simulink model "stm32f0_ccp_sensor"  (Simulink 7.3)
settings: Solver=ode3  SolverMode=SingleTasking  StartTime=0.0  StopTime=10.0  RelTol=1e-3
PreLoadFcn:
  | waijung.modelPreload; % Required for working with Waijung Blockset. Do not remove.
undefined symbols (not defined in the file): ARM, LQFP48, MDK, STM32F072CB
libraries: simulink x216, waijung_soft_i2c_lib x28, waijung_addon_module x12, stm32f0_flash_lib x10, stm32f0_can_lib x3, stm32f0_reset_lib x1, waijung_crc_lib x1, stm32f0_boot_lib x1, stm32f0_device_config_lib x1
(part 5 of 6)

== system stm32f0_ccp_sensor/CCP Handler/Command Processing/BUILD_CHKSUM/BUILD_CHKSUM Handler/Subsystem/While Iterator Subsystem ==
  Address : Inport  OutDataType=fixdt(1, 16)  OutScaling=2^0
  Size : Inport  Port=2  OutDataType=fixdt(1, 16)  OutScaling=2^0
  Add : Sum  OutDataType=fixdt(1, 16)  OutScaling=2^-10
  Add1 : Sum  OutDataType=fixdt(1, 16)  OutScaling=2^-10
  Bitwise Operator : simulink/Logic and Bit Operations/Bitwise Operator  logicop=AND  UseBitMask=on  BitMask=hex2dec('01FFFFFF')  BitMaskRealWorld=Stored Integer
  Bitwise Operator1 : simulink/Logic and Bit Operations/Bitwise Operator  logicop=AND  UseBitMask=on  BitMask=hex2dec('0001FFFF')  BitMaskRealWorld=Stored Integer
  Compare To Zero : simulink/Logic and Bit Operations/Compare To Zero  SystemSampleTime=-1  relop===  LogicOutDataTypeMode=uint8  ZeroCross=off
  Initial : Constant  Value=0  OutDataTypeMode=uint32  OutDataType=fixdt(1, 16)  OutScaling=2^0  OutDataTypeStr=uint32
  Initial1 : Constant  Value=hex2dec('FFFFFFFF')  OutDataTypeMode=uint32  OutDataType=fixdt(1, 16)  OutScaling=2^0  OutDataTypeStr=uint32
  Memory : Memory  InheritSampleTime=on  LinearizeMemory=on
  Memory1 : Memory  InheritSampleTime=on  LinearizeMemory=on
  Relational Operator : RelationalOperator  Operator=>  LogicOutDataTypeMode=boolean  LogicDataType=fixdt(0, 8)  OutDataTypeStr=boolean
  Step : Constant  Value=4  OutDataTypeMode=uint32  OutDataType=fixdt(1, 16)  OutScaling=2^0  OutDataTypeStr=uint32
  Subsystem : Subsystem
  Switch : Switch  Criteria=u2 ~= 0  OutDataType=fixdt(1, 16)  OutScaling=2^0
  Switch1 : Switch  Criteria=u2 ~= 0  OutDataType=fixdt(1, 16)  OutScaling=2^0
  While Iterator : WhileIterator  MaxIters=-1  WhileBlockType=do-while
  CRC : Outport  OutDataType=fixdt(1, 16)  OutScaling=2^0
  wires:
  Initial/1 -> Switch/3
  Add1/1 -> Switch/1
  Relational Operator/1 -> Switch/2, While Iterator/1, Subsystem/Enable
  Switch/1 -> Memory/1
  Size/1 -> Relational Operator/1
  Step/1 -> Add1/2
  Add/1 -> Bitwise Operator/1
  Memory/1 -> Add/2, Relational Operator/2, Add1/1, Compare To Zero/1
  Address/1 -> Bitwise Operator1/1
  Compare To Zero/1 -> Switch1/2
  Initial1/1 -> Switch1/1
  Switch1/1 -> Subsystem/1(In1)
  Subsystem/1(Out1) -> Memory1/1, CRC/1
  Memory1/1 -> Switch1/3
  Bitwise Operator/1 -> Subsystem/2(In2)
  Bitwise Operator1/1 -> Add/1

== system stm32f0_ccp_sensor/CCP Handler/Command Processing/CLEAR_MEMORY/CLEAR_MEMORY Handler/Flash Erase/While Iterator Subsystem ==
  Address : Inport  OutDataType=fixdt(1, 16)  OutScaling=2^0
  Size : Inport  Port=2  OutDataType=fixdt(1, 16)  OutScaling=2^0
  Add : Sum  OutDataType=fixdt(1, 16)  OutScaling=2^-10
  Add1 : Sum  OutDataType=fixdt(1, 16)  OutScaling=2^-10
  Bitwise Operator : simulink/Logic and Bit Operations/Bitwise Operator  logicop=AND  UseBitMask=on  BitMask=hex2dec('0000FFFF')  BitMaskRealWorld=Stored Integer
  Initial : Constant  Value=0  OutDataTypeMode=uint32  OutDataType=fixdt(1, 16)  OutScaling=2^0  OutDataTypeStr=uint32
  Memory : Memory  InheritSampleTime=on  LinearizeMemory=on
  Relational Operator : RelationalOperator  Operator=>  LogicOutDataTypeMode=boolean  LogicDataType=fixdt(0, 8)  OutDataTypeStr=boolean
  Step : Constant  Value=2048  OutDataTypeMode=uint32  OutDataType=fixdt(1, 16)  OutScaling=2^0  OutDataTypeStr=uint32
  Subsystem : Subsystem
  Switch : Switch  Criteria=u2 ~= 0  OutDataType=fixdt(1, 16)  OutScaling=2^0
  While Iterator : WhileIterator  MaxIters=-1  WhileBlockType=do-while
  Sta : Outport  OutDataType=fixdt(1, 16)  OutScaling=2^0
  wires:
  Bitwise Operator/1 -> Subsystem/1(Address)
  Subsystem/1(Sta) -> Sta/1
  Address/1 -> Add/1
  Memory/1 -> Add1/1, Relational Operator/2, Add/2
  Add/1 -> Bitwise Operator/1
  Step/1 -> Add1/2
  Size/1 -> Relational Operator/1
  Switch/1 -> Memory/1
  Relational Operator/1 -> Switch/2, While Iterator/1, Subsystem/Enable
  Add1/1 -> Switch/1
  Initial/1 -> Switch/3

== system stm32f0_ccp_sensor/CCP Handler/Command Processing/PROGRAM/ PROGRAM_6/PROGRAM/PROGRAM_6 Handler/EEPROM Program/Subsystem ==
  SlaveAddr : Inport
  Offset : Inport  Port=2
  D0 : Inport  Port=3
  Enable : EnablePort
  Compare To Zero : simulink/Logic and Bit Operations/Compare To Zero  SystemSampleTime=-1  relop===  LogicOutDataTypeMode=uint8  ZeroCross=off
  Soft I2C Master Read/Write : waijung_soft_i2c_lib/Soft I2C Master Read//Write  conf=ReadWrite  targetname=stm32f0  module=1  transfer=Blocking  clk=100  timeout=25  sdapins={'A4','A6'}  sclpins='A5'  writecount=2  readcount=0  waittime=5  forcestop=off  portpinstr=0  sampletime=inf  blockid=CCPHandlerCommandProcessingPROGRAMPROGRAM_6PROGRAMPROGRAM_6HandlerEEPROMProgramSubsystemSoftI2CMasterReadWrite  inputporttype=[3 3 3]  inputportwidth=[]  inputportlabel={'SlvAddr' 'Wr0 (uint8)' 'Wr1 (uint8)'}  outputporttype=[3]  outputportwidth=[1]  outputportlabel={'Status'}  compat=0  optionstring="[\"1\",\"2\",\"0\",\"5\",\"off\",\"1\"]"
  Success : Outport
  wires:
  SlaveAddr/1 -> Soft I2C Master Read/Write/1
  Offset/1 -> Soft I2C Master Read/Write/2
  Soft I2C Master Read/Write/1 -> Compare To Zero/1
  D0/1 -> Soft I2C Master Read/Write/3
  Compare To Zero/1 -> Success/1

== system stm32f0_ccp_sensor/CCP Handler/Command Processing/PROGRAM/ PROGRAM_6/PROGRAM/PROGRAM_6 Handler/EEPROM Program/Subsystem1 ==
  SlaveAddr : Inport
  Offset : Inport  Port=2
  D0 : Inport  Port=3
  D1 : Inport  Port=4
  Enable : EnablePort
  Compare To Zero : simulink/Logic and Bit Operations/Compare To Zero  SystemSampleTime=-1  relop===  LogicOutDataTypeMode=uint8  ZeroCross=off
  Soft I2C Master Read/Write : waijung_soft_i2c_lib/Soft I2C Master Read//Write  conf=ReadWrite  targetname=stm32f0  module=1  transfer=Blocking  clk=100  timeout=25  sdapins={'A4','A6'}  sclpins='A5'  writecount=3  readcount=0  waittime=5  forcestop=off  portpinstr=0  sampletime=inf  blockid=CCPHandlerCommandProcessingPROGRAMPROGRAM_6PROGRAMPROGRAM_6HandlerEEPROMProgramSubsystem1SoftI2CMasterReadWrite  inputporttype=[3 3 3 3]  inputportwidth=[]  inputportlabel={'SlvAddr' 'Wr0 (uint8)' 'Wr1 (uint8)' 'Wr2 (uint8)'}  outputporttype=[3]  outputportwidth=[1]  outputportlabel={'Status'}  compat=0  optionstring="[\"1\",\"3\",\"0\",\"5\",\"off\",\"1\"]"
  Success : Outport
  wires:
  Compare To Zero/1 -> Success/1
  D0/1 -> Soft I2C Master Read/Write/3
  Soft I2C Master Read/Write/1 -> Compare To Zero/1
  Offset/1 -> Soft I2C Master Read/Write/2
  SlaveAddr/1 -> Soft I2C Master Read/Write/1
  D1/1 -> Soft I2C Master Read/Write/4

== system stm32f0_ccp_sensor/CCP Handler/Command Processing/PROGRAM/ PROGRAM_6/PROGRAM/PROGRAM_6 Handler/EEPROM Program/Subsystem2 ==
  SlaveAddr : Inport
  Offset : Inport  Port=2
  D0 : Inport  Port=3
  D1 : Inport  Port=4
  D2 : Inport  Port=5
  Enable : EnablePort
  Compare To Zero : simulink/Logic and Bit Operations/Compare To Zero  SystemSampleTime=-1  relop===  LogicOutDataTypeMode=uint8  ZeroCross=off
  Soft I2C Master Read/Write : waijung_soft_i2c_lib/Soft I2C Master Read//Write  conf=ReadWrite  targetname=stm32f0  module=1  transfer=Blocking  clk=100  timeout=25  sdapins={'A4','A6'}  sclpins='A5'  writecount=4  readcount=0  waittime=5  forcestop=off  portpinstr=0  sampletime=inf  blockid=CCPHandlerCommandProcessingPROGRAMPROGRAM_6PROGRAMPROGRAM_6HandlerEEPROMProgramSubsystem2SoftI2CMasterReadWrite  inputporttype=[3 3 3 3 3]  inputportwidth=[]  inputportlabel={'SlvAddr' 'Wr0 (uint8)' 'Wr1 (uint8)' 'Wr2 (uint8)' 'Wr3 (uint8)'}  outputporttype=[3]  outputportwidth=[1]  outputportlabel={'Status'}  compat=0  optionstring="[\"1\",\"4\",\"0\",\"5\",\"off\",\"1\"]"
  Success : Outport
  wires:
  D1/1 -> Soft I2C Master Read/Write/4
  SlaveAddr/1 -> Soft I2C Master Read/Write/1
  Offset/1 -> Soft I2C Master Read/Write/2
  Soft I2C Master Read/Write/1 -> Compare To Zero/1
  D0/1 -> Soft I2C Master Read/Write/3
  Compare To Zero/1 -> Success/1
  D2/1 -> Soft I2C Master Read/Write/5

== system stm32f0_ccp_sensor/CCP Handler/Command Processing/PROGRAM/ PROGRAM_6/PROGRAM/PROGRAM_6 Handler/EEPROM Program/Subsystem3 ==
  SlaveAddr : Inport
  Offset : Inport  Port=2
  D0 : Inport  Port=3
  D1 : Inport  Port=4
  D2 : Inport  Port=5
  D3 : Inport  Port=6
  Enable : EnablePort
  Compare To Zero : simulink/Logic and Bit Operations/Compare To Zero  SystemSampleTime=-1  relop===  LogicOutDataTypeMode=uint8  ZeroCross=off
  Soft I2C Master Read/Write : waijung_soft_i2c_lib/Soft I2C Master Read//Write  conf=ReadWrite  targetname=stm32f0  module=1  transfer=Blocking  clk=100  timeout=25  sdapins={'A4','A6'}  sclpins='A5'  writecount=5  readcount=0  waittime=5  forcestop=off  portpinstr=0  sampletime=inf  blockid=CCPHandlerCommandProcessingPROGRAMPROGRAM_6PROGRAMPROGRAM_6HandlerEEPROMProgramSubsystem3SoftI2CMasterReadWrite  inputporttype=[3 3 3 3 3 3]  inputportwidth=[]  inputportlabel={'SlvAddr' 'Wr0 (uint8)' 'Wr1 (uint8)' 'Wr2 (uint8)' 'Wr3 (uint8)' 'Wr4 (uint8)'}  outputporttype=[3]  outputportwidth=[1]  outputportlabel={'Status'}  compat=0  optionstring="[\"1\",\"5\",\"0\",\"5\",\"off\",\"1\"]"
  Success : Outport
  wires:
  D2/1 -> Soft I2C Master Read/Write/5
  Compare To Zero/1 -> Success/1
  D0/1 -> Soft I2C Master Read/Write/3
  Soft I2C Master Read/Write/1 -> Compare To Zero/1
  Offset/1 -> Soft I2C Master Read/Write/2
  SlaveAddr/1 -> Soft I2C Master Read/Write/1
  D1/1 -> Soft I2C Master Read/Write/4
  D3/1 -> Soft I2C Master Read/Write/6

== system stm32f0_ccp_sensor/CCP Handler/Command Processing/PROGRAM/ PROGRAM_6/PROGRAM/PROGRAM_6 Handler/EEPROM Program/Subsystem4 ==
  SlaveAddr : Inport
  Offset : Inport  Port=2
  D0 : Inport  Port=3
  D1 : Inport  Port=4
  D2 : Inport  Port=5
  D3 : Inport  Port=6
  D4 : Inport  Port=7
  Enable : EnablePort
  Compare To Zero : simulink/Logic and Bit Operations/Compare To Zero  SystemSampleTime=-1  relop===  LogicOutDataTypeMode=uint8  ZeroCross=off
  Soft I2C Master Read/Write : waijung_soft_i2c_lib/Soft I2C Master Read//Write  conf=ReadWrite  targetname=stm32f0  module=1  transfer=Blocking  clk=100  timeout=25  sdapins={'A4','A6'}  sclpins='A5'  writecount=6  readcount=0  waittime=5  forcestop=off  portpinstr=0  sampletime=inf  blockid=CCPHandlerCommandProcessingPROGRAMPROGRAM_6PROGRAMPROGRAM_6HandlerEEPROMProgramSubsystem4SoftI2CMasterReadWrite  inputporttype=[3 3 3 3 3 3 3]  inputportwidth=[]  inputportlabel={'SlvAddr' 'Wr0 (uint8)' 'Wr1 (uint8)' 'Wr2 (uint8)' 'Wr3 (uint8)' 'Wr4 (uint8)' 'Wr5 (uint8)'}  outputporttype=[3]  outputportwidth=[1]  outputportlabel={'Status'}  compat=0  optionstring="[\"1\",\"6\",\"0\",\"5\",\"off\",\"1\"]"
  Success : Outport
  wires:
  D3/1 -> Soft I2C Master Read/Write/6
  D1/1 -> Soft I2C Master Read/Write/4
  SlaveAddr/1 -> Soft I2C Master Read/Write/1
  Offset/1 -> Soft I2C Master Read/Write/2
  Soft I2C Master Read/Write/1 -> Compare To Zero/1
  D0/1 -> Soft I2C Master Read/Write/3
  Compare To Zero/1 -> Success/1
  D2/1 -> Soft I2C Master Read/Write/5
  D4/1 -> Soft I2C Master Read/Write/7

== system stm32f0_ccp_sensor/CCP Handler/Command Processing/PROGRAM/ PROGRAM_6/PROGRAM/PROGRAM_6 Handler/Flash Program/Subsystem ==
  Addr : Inport
  In3 : Inport  Port=2
  In4 : Inport  Port=3
  Enable : EnablePort
  Bitwise Operator : simulink/Logic and Bit Operations/Bitwise Operator  logicop=OR  UseBitMask=off  NumInputPorts=2  BitMask=bin2dec('11011001')  BitMaskRealWorld=Stored Integer
  Data Type Conversion : DataTypeConversion  OutDataTypeMode=uint16  OutDataType=fixdt(1, 16)  OutScaling=2^0  OutDataTypeStr=uint16
  Data Type Conversion1 : DataTypeConversion  OutDataTypeMode=uint16  OutDataType=fixdt(1, 16)  OutScaling=2^0  OutDataTypeStr=uint16
  FLASH Write : stm32f0_flash_lib/FLASH Write  conf=Write  startaddress=0x8011000  pagesize=2k  datatype=uint16  enablestatus=on  sampletime=inf  filename='stm32f0_ccp_sensor.flash'  enablecustomportlabel=off  cinputportlabel=0  portpinstr=0  blockid=CCPHandlerCommandProcessingPROGRAMPROGRAM_6PROGRAMPROGRAM_6HandlerFlashProgramSubsystemFLASHWrite  inputporttype=[7 5]  inputportwidth=[]  inputportlabel={'Offset','Data (uint16)'}  outputporttype=[3]  outputportwidth=[]  outputportlabel={'Status'}  compat=0  optionstring="[\"8011000\",\"0\"]"
  FLASH_COMPLETE : simulink/Logic and Bit Operations/Compare To Constant  SystemSampleTime=-1  relop===  const=4  LogicOutDataTypeMode=uint8  ZeroCross=off
  Shift Arithmetic : simulink/Logic and Bit Operations/Shift Arithmetic  SystemSampleTime=-1  nBitShiftRight=-8  nBinPtShiftRight=0
  Success : Outport
  wires:
  In3/1 -> Data Type Conversion/1
  In4/1 -> Data Type Conversion1/1
  Data Type Conversion1/1 -> Shift Arithmetic/1
  Shift Arithmetic/1 -> Bitwise Operator/2
  Data Type Conversion/1 -> Bitwise Operator/1
  Bitwise Operator/1 -> FLASH Write/2
  Addr/1 -> FLASH Write/1
  FLASH Write/1 -> FLASH_COMPLETE/1
  FLASH_COMPLETE/1 -> Success/1

== system stm32f0_ccp_sensor/CCP Handler/Command Processing/PROGRAM/ PROGRAM_6/PROGRAM/PROGRAM_6 Handler/Flash Program/Subsystem1 ==
  Addr : Inport
  In3 : Inport  Port=2
  In4 : Inport  Port=3
  In1 : Inport  Port=4
  In2 : Inport  Port=5
  Enable : EnablePort
  Bitwise Operator : simulink/Logic and Bit Operations/Bitwise Operator  logicop=OR  UseBitMask=off  NumInputPorts=4  BitMask=bin2dec('11011001')  BitMaskRealWorld=Stored Integer
  Data Type Conversion{,1..3} (4 alike) : DataTypeConversion  OutDataTypeMode=uint32  OutDataType=fixdt(1, 16)  OutScaling=2^0  OutDataTypeStr=uint32
  FLASH Write : stm32f0_flash_lib/FLASH Write  conf=Write  startaddress=0x8011000  pagesize=2k  datatype=uint32  enablestatus=on  sampletime=inf  filename='stm32f0_ccp_sensor.flash'  enablecustomportlabel=off  cinputportlabel=0  portpinstr=0  blockid=CCPHandlerCommandProcessingPROGRAMPROGRAM_6PROGRAMPROGRAM_6HandlerFlashProgramSubsystem1FLASHWrite  inputporttype=[7 7]  inputportwidth=[]  inputportlabel={'Offset','Data (uint32)'}  outputporttype=[3]  outputportwidth=[]  outputportlabel={'Status'}  compat=0  optionstring="[\"8011000\",\"0\"]"
  FLASH_COMPLETE : simulink/Logic and Bit Operations/Compare To Constant  SystemSampleTime=-1  relop===  const=4  LogicOutDataTypeMode=uint8  ZeroCross=off
  Shift Arithmetic : simulink/Logic and Bit Operations/Shift Arithmetic  SystemSampleTime=-1  nBitShiftRight=-8  nBinPtShiftRight=0
  Shift Arithmetic1 : simulink/Logic and Bit Operations/Shift Arithmetic  SystemSampleTime=-1  nBitShiftRight=-16  nBinPtShiftRight=0
  Shift Arithmetic2 : simulink/Logic and Bit Operations/Shift Arithmetic  SystemSampleTime=-1  nBitShiftRight=-24  nBinPtShiftRight=0
  Success : Outport
  wires:
  Bitwise Operator/1 -> FLASH Write/2
  Addr/1 -> FLASH Write/1
  Data Type Conversion/1 -> Bitwise Operator/1
  Shift Arithmetic/1 -> Bitwise Operator/2
  Data Type Conversion1/1 -> Shift Arithmetic/1
  In4/1 -> Data Type Conversion1/1
  In3/1 -> Data Type Conversion/1
  In1/1 -> Data Type Conversion2/1
  In2/1 -> Data Type Conversion3/1
  Data Type Conversion2/1 -> Shift Arithmetic1/1
  Data Type Conversion3/1 -> Shift Arithmetic2/1
  Shift Arithmetic1/1 -> Bitwise Operator/3
  Shift Arithmetic2/1 -> Bitwise Operator/4
  FLASH Write/1 -> FLASH_COMPLETE/1
  FLASH_COMPLETE/1 -> Success/1

== system stm32f0_ccp_sensor/CCP Handler/Command Processing/PROGRAM/ PROGRAM_6/PROGRAM/PROGRAM_6 Handler/Flash Program 6/Subsystem ==
  In1 : Inport
  In2 : Inport  Port=2
  Bitwise Operator : simulink/Logic and Bit Operations/Bitwise Operator  logicop=OR  UseBitMask=off  NumInputPorts=2  BitMask=bin2dec('11011001')  BitMaskRealWorld=Stored Integer
  Data Type Conversion : DataTypeConversion  OutDataTypeMode=uint16  OutDataType=fixdt(1, 16)  OutScaling=2^0  OutDataTypeStr=uint16
  Data Type Conversion1 : DataTypeConversion  OutDataTypeMode=uint16  OutDataType=fixdt(1, 16)  OutScaling=2^0  OutDataTypeStr=uint16
  Shift Arithmetic : simulink/Logic and Bit Operations/Shift Arithmetic  SystemSampleTime=-1  nBitShiftRight=-8  nBinPtShiftRight=0
  Out1 : Outport
  wires:
  Data Type Conversion1/1 -> Shift Arithmetic/1
  Shift Arithmetic/1 -> Bitwise Operator/2
  Data Type Conversion/1 -> Bitwise Operator/1
  In1/1 -> Data Type Conversion/1
  Bitwise Operator/1 -> Out1/1
  In2/1 -> Data Type Conversion1/1

== system stm32f0_ccp_sensor/CCP Handler/Command Processing/PROGRAM/ PROGRAM_6/PROGRAM/PROGRAM_6 Handler/Flash Program 6/Subsystem1 ==
  In1 : Inport
  In2 : Inport  Port=2
  In3 : Inport  Port=3
  In4 : Inport  Port=4
  Bitwise Operator : simulink/Logic and Bit Operations/Bitwise Operator  logicop=OR  UseBitMask=off  NumInputPorts=4  BitMask=bin2dec('11011001')  BitMaskRealWorld=Stored Integer
  Data Type Conversion{,1..3} (4 alike) : DataTypeConversion  OutDataTypeMode=uint32  OutDataType=fixdt(1, 16)  OutScaling=2^0  OutDataTypeStr=uint32
  Shift Arithmetic : simulink/Logic and Bit Operations/Shift Arithmetic  SystemSampleTime=-1  nBitShiftRight=-8  nBinPtShiftRight=0
  Shift Arithmetic1 : simulink/Logic and Bit Operations/Shift Arithmetic  SystemSampleTime=-1  nBitShiftRight=-16  nBinPtShiftRight=0
  Shift Arithmetic2 : simulink/Logic and Bit Operations/Shift Arithmetic  SystemSampleTime=-1  nBitShiftRight=-24  nBinPtShiftRight=0
  Out1 : Outport
  wires:
  Data Type Conversion/1 -> Bitwise Operator/1
  Shift Arithmetic/1 -> Bitwise Operator/2
  Data Type Conversion1/1 -> Shift Arithmetic/1
  Data Type Conversion2/1 -> Shift Arithmetic1/1
  Data Type Conversion3/1 -> Shift Arithmetic2/1
  Shift Arithmetic1/1 -> Bitwise Operator/3
  Shift Arithmetic2/1 -> Bitwise Operator/4
  In1/1 -> Data Type Conversion/1
  Bitwise Operator/1 -> Out1/1
  In2/1 -> Data Type Conversion1/1
  In3/1 -> Data Type Conversion2/1
  In4/1 -> Data Type Conversion3/1

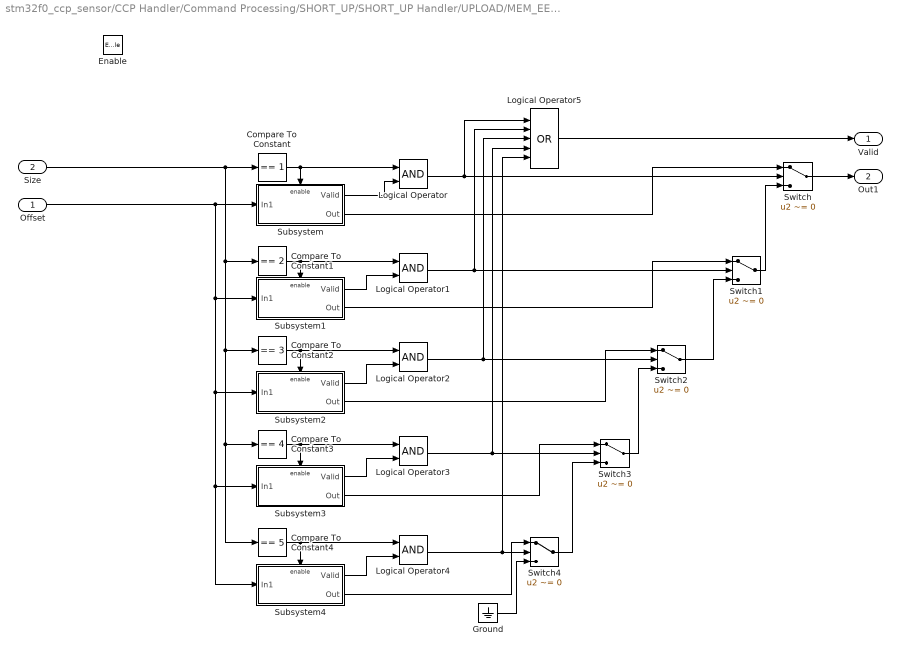
== system stm32f0_ccp_sensor/CCP Handler/Command Processing/SHORT_UP/SHORT_UP Handler/UPLOAD/MEM_EEPROM ==
  Offset : Inport  OutDataType=fixdt(1, 16)  OutScaling=2^0
  Size : Inport  Port=2  OutDataType=fixdt(1, 16)  OutScaling=2^0
  Enable : EnablePort
  Compare To Constant : simulink/Logic and Bit Operations/Compare To Constant  SystemSampleTime=-1  relop===  const=1  LogicOutDataTypeMode=uint8  ZeroCross=off
  Compare To Constant1 : simulink/Logic and Bit Operations/Compare To Constant  SystemSampleTime=-1  relop===  const=2  LogicOutDataTypeMode=uint8  ZeroCross=off
  Compare To Constant2 : simulink/Logic and Bit Operations/Compare To Constant  SystemSampleTime=-1  relop===  const=3  LogicOutDataTypeMode=uint8  ZeroCross=off
  Compare To Constant3 : simulink/Logic and Bit Operations/Compare To Constant  SystemSampleTime=-1  relop===  const=4  LogicOutDataTypeMode=uint8  ZeroCross=off
  Compare To Constant4 : simulink/Logic and Bit Operations/Compare To Constant  SystemSampleTime=-1  relop===  const=5  LogicOutDataTypeMode=uint8  ZeroCross=off
  Ground : Ground
  Logical Operator{,1..4} (5 alike) : Logic  AllPortsSameDT=off  OutDataTypeMode=boolean  LogicDataType=fixdt(0, 8)  OutDataTypeStr=boolean
  Logical Operator5 : Logic  Operator=OR  Inputs=5  AllPortsSameDT=off  OutDataTypeMode=boolean  LogicDataType=fixdt(0, 8)  OutDataTypeStr=boolean
  Subsystem : Subsystem
  Subsystem1 : Subsystem
  Subsystem2 : Subsystem
  Subsystem3 : Subsystem
  Subsystem4 : Subsystem
  Switch{,1..4} (5 alike) : Switch  Criteria=u2 ~= 0  OutDataType=fixdt(1, 16)  OutScaling=2^0
  Valid : Outport  OutDataType=fixdt(1, 16)  OutScaling=2^0
  Out1 : Outport  Port=2  OutDataType=fixdt(1, 16)  OutScaling=2^0
  wires:
  Offset/1 -> Subsystem/1(In1), Subsystem1/1(In1), Subsystem2/1(In1), Subsystem3/1(In1), Subsystem4/1(In1)
  Compare To Constant/1 -> Subsystem/Enable, Logical Operator/1
  Size/1 -> Compare To Constant/1, Compare To Constant1/1, Compare To Constant2/1, Compare To Constant3/1, Compare To Constant4/1
  Compare To Constant1/1 -> Subsystem1/Enable, Logical Operator1/1
  Compare To Constant2/1 -> Subsystem2/Enable, Logical Operator2/1
  Compare To Constant3/1 -> Subsystem3/Enable, Logical Operator3/1
  Compare To Constant4/1 -> Subsystem4/Enable, Logical Operator4/1
  Subsystem/1(Valid) -> Logical Operator/2
  Subsystem1/1(Valid) -> Logical Operator1/2
  Subsystem2/1(Valid) -> Logical Operator2/2
  Subsystem3/1(Valid) -> Logical Operator3/2
  Subsystem4/1(Valid) -> Logical Operator4/2
  Logical Operator5/1 -> Valid/1
  Logical Operator/1 -> Logical Operator5/1, Switch/2
  Logical Operator4/1 -> Logical Operator5/5, Switch4/2
  Logical Operator3/1 -> Logical Operator5/4, Switch3/2
  Logical Operator2/1 -> Logical Operator5/3, Switch2/2
  Logical Operator1/1 -> Logical Operator5/2, Switch1/2
  Subsystem/2(Out) -> Switch/1
  Subsystem1/2(Out) -> Switch1/1
  Switch1/1 -> Switch/3
  Subsystem2/2(Out) -> Switch2/1
  Switch2/1 -> Switch1/3
  Switch/1 -> Out1/1
  Subsystem3/2(Out) -> Switch3/1
  Switch3/1 -> Switch2/3
  Switch4/1 -> Switch3/3
  Subsystem4/2(Out) -> Switch4/1
  Ground/1 -> Switch4/3

== system stm32f0_ccp_sensor/CCP Handler/Command Processing/SHORT_UP/SHORT_UP Handler/UPLOAD/MEM_FLASH ==
  Offset : Inport  OutDataType=fixdt(1, 16)  OutScaling=2^0
  Size : Inport  Port=2  OutDataType=fixdt(1, 16)  OutScaling=2^0
  Enable : EnablePort
  Compare To Constant : simulink/Logic and Bit Operations/Compare To Constant  SystemSampleTime=-1  relop===  const=2  LogicOutDataTypeMode=uint8  ZeroCross=off
  Compare To Constant1 : simulink/Logic and Bit Operations/Compare To Constant  SystemSampleTime=-1  relop===  const=4  LogicOutDataTypeMode=uint8  ZeroCross=off
  Logical Operator : Logic  Operator=OR  AllPortsSameDT=off  OutDataTypeMode=boolean  LogicDataType=fixdt(0, 8)  OutDataTypeStr=boolean
  Read Flash 2 Byte : Subsystem  TreatAsAtomicUnit=on
  Read Flash 4 Byte : Subsystem  TreatAsAtomicUnit=on
  Switch : Switch  OutDataType=fixdt(1, 16)  OutScaling=2^0
  Valid : Outport  OutDataType=fixdt(1, 16)  OutScaling=2^0
  Out1 : Outport  Port=2  OutDataType=fixdt(1, 16)  OutScaling=2^0
  wires:
  Logical Operator/1 -> Valid/1
  Size/1 -> Compare To Constant/1, Compare To Constant1/1
  Compare To Constant/1 -> Read Flash 2 Byte/Enable, Logical Operator/1, Switch/2
  Compare To Constant1/1 -> Read Flash 4 Byte/Enable, Logical Operator/2
  Offset/1 -> Read Flash 2 Byte/1(Offset), Read Flash 4 Byte/1(In1)
  Read Flash 2 Byte/1(Out1) -> Switch/1
  Read Flash 4 Byte/1(Out1) -> Switch/3
  Switch/1 -> Out1/1

== system stm32f0_ccp_sensor/CCP Handler/Command Processing/SHORT_UP/SHORT_UP Handler/UPLOAD/MEM_RO ==
  Offset : Inport  OutDataType=fixdt(1, 16)  OutScaling=2^0
  Size : Inport  Port=2  OutDataType=fixdt(1, 16)  OutScaling=2^0
  Enable : EnablePort
  Constant : Constant  OutDataTypeMode=uint8  OutDataType=fixdt(1, 16)  OutScaling=2^0  OutDataTypeStr=uint8
  Volatile Data Array Read : waijung_addon_module/Data Storage/Volatile Data Array Read  conf=Read  specificaddress=off  storagename=READ_DATA  memoryaddress=hex2dec('64000000')  storagetype=uint8  datasize=120*160*3  varname=VolatileDataArray_READ_DATA  datatype=uint8  datacount=5  variablesize=on  portpinstr=0  sampletime=inf  blockid=CCPHandlerCommandProcessingSHORT_UPSHORT_UPHandlerUPLOADMEM_ROVolatileDataArrayRead  inputporttype=[7 7]  inputportwidth=[1 1 ]  inputportlabel={'Offset','Size'}  outputporttype=[3]  outputportwidth=[5]  outputportlabel={'Data(5)'}  compat=0  optionstring="[\"READ_DATA\",\"uint8\",\"256\",\"VolatileDataArray_READ_DATA\",\"uint8_t\",\"uint8\",\"uint8_t\",\"5\",\"Param1\"]"
  Valid : Outport  OutDataType=fixdt(1, 16)  OutScaling=2^0
  Out1 : Outport  Port=2  OutDataType=fixdt(1, 16)  OutScaling=2^0
  wires:
  Offset/1 -> Volatile Data Array Read/1
  Volatile Data Array Read/1 -> Out1/1
  Size/1 -> Volatile Data Array Read/2
  Constant/1 -> Valid/1

== system stm32f0_ccp_sensor/CCP Handler/Command Processing/SHORT_UP/SHORT_UP Handler/UPLOAD/MEM_RW ==
  Offset : Inport  OutDataType=fixdt(1, 16)  OutScaling=2^0
  Size : Inport  Port=2  OutDataType=fixdt(1, 16)  OutScaling=2^0
  Enable : EnablePort
  Constant : Constant  OutDataTypeMode=uint8  OutDataType=fixdt(1, 16)  OutScaling=2^0  OutDataTypeStr=uint8
  Volatile Data Array Read : waijung_addon_module/Data Storage/Volatile Data Array Read  conf=Read  specificaddress=off  storagename=CONTROL  memoryaddress=hex2dec('64000000')  storagetype=uint8  datasize=120*160*3  varname=VolatileDataArray_CONTROL  datatype=uint8  datacount=5  variablesize=on  portpinstr=0  sampletime=inf  blockid=CCPHandlerCommandProcessingSHORT_UPSHORT_UPHandlerUPLOADMEM_RWVolatileDataArrayRead  inputporttype=[7 7]  inputportwidth=[1 1 ]  inputportlabel={'Offset','Size'}  outputporttype=[3]  outputportwidth=[5]  outputportlabel={'Data(5)'}  compat=0  optionstring="[\"CONTROL\",\"uint8\",\"256\",\"VolatileDataArray_CONTROL\",\"uint8_t\",\"uint8\",\"uint8_t\",\"5\",\"Param1\"]"
  Valid : Outport  OutDataType=fixdt(1, 16)  OutScaling=2^0
  Out1 : Outport  Port=2  OutDataType=fixdt(1, 16)  OutScaling=2^0
  wires:
  Offset/1 -> Volatile Data Array Read/1
  Size/1 -> Volatile Data Array Read/2
  Volatile Data Array Read/1 -> Out1/1
  Constant/1 -> Valid/1

== system stm32f0_ccp_sensor/CCP Handler/Command Processing/SHORT_UP/SHORT_UP Handler/UPLOAD/SLAVE_DEVICE_ID ==
  Offset : Inport  OutDataType=fixdt(1, 16)  OutScaling=2^0
  Size : Inport  Port=2  OutDataType=fixdt(1, 16)  OutScaling=2^0
  Enable : EnablePort
  Constant : Constant  OutDataTypeMode=uint8  OutDataType=fixdt(1, 16)  OutScaling=2^0  OutDataTypeStr=uint8
  Volatile Data Array Read : waijung_addon_module/Data Storage/Volatile Data Array Read  conf=Read  specificaddress=off  storagename=SLAVE_DEV_ID  memoryaddress=hex2dec('64000000')  storagetype=uint8  datasize=120*160*3  varname=VolatileDataArray_SLAVE_DEV_ID  datatype=uint8  datacount=5  variablesize=on  portpinstr=0  sampletime=inf  blockid=CCPHandlerCommandProcessingSHORT_UPSHORT_UPHandlerUPLOADSLAVE_DEVICE_IDVolatileDataArrayRead  inputporttype=[7 7]  inputportwidth=[1 1 ]  inputportlabel={'Offset','Size'}  outputporttype=[3]  outputportwidth=[5]  outputportlabel={'Data(5)'}  compat=0  optionstring="[\"SLAVE_DEV_ID\",\"uint8\",\"16\",\"VolatileDataArray_SLAVE_DEV_ID\",\"uint8_t\",\"uint8\",\"uint8_t\",\"5\",\"Param1\"]"
  Valid : Outport  OutDataType=fixdt(1, 16)  OutScaling=2^0
  Out1 : Outport  Port=2  OutDataType=fixdt(1, 16)  OutScaling=2^0
  wires:
  Offset/1 -> Volatile Data Array Read/1
  Size/1 -> Volatile Data Array Read/2
  Volatile Data Array Read/1 -> Out1/1
  Constant/1 -> Valid/1

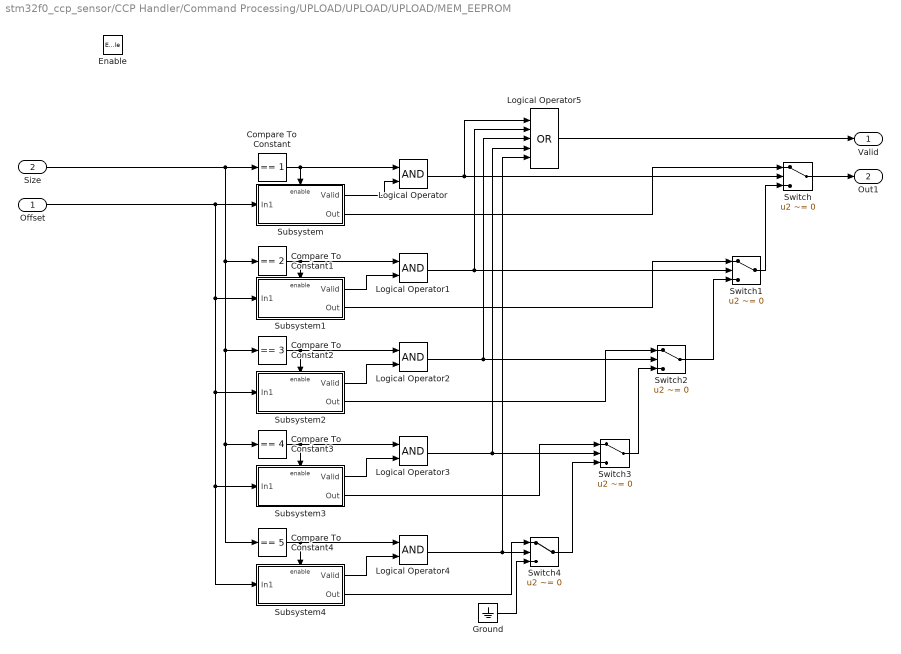
== system stm32f0_ccp_sensor/CCP Handler/Command Processing/UPLOAD/UPLOAD/UPLOAD/MEM_EEPROM ==
  Offset : Inport  OutDataType=fixdt(1, 16)  OutScaling=2^0
  Size : Inport  Port=2  OutDataType=fixdt(1, 16)  OutScaling=2^0
  Enable : EnablePort
  Compare To Constant : simulink/Logic and Bit Operations/Compare To Constant  SystemSampleTime=-1  relop===  const=1  LogicOutDataTypeMode=uint8  ZeroCross=off
  Compare To Constant1 : simulink/Logic and Bit Operations/Compare To Constant  SystemSampleTime=-1  relop===  const=2  LogicOutDataTypeMode=uint8  ZeroCross=off
  Compare To Constant2 : simulink/Logic and Bit Operations/Compare To Constant  SystemSampleTime=-1  relop===  const=3  LogicOutDataTypeMode=uint8  ZeroCross=off
  Compare To Constant3 : simulink/Logic and Bit Operations/Compare To Constant  SystemSampleTime=-1  relop===  const=4  LogicOutDataTypeMode=uint8  ZeroCross=off
  Compare To Constant4 : simulink/Logic and Bit Operations/Compare To Constant  SystemSampleTime=-1  relop===  const=5  LogicOutDataTypeMode=uint8  ZeroCross=off
  Ground : Ground
  Logical Operator{,1..4} (5 alike) : Logic  AllPortsSameDT=off  OutDataTypeMode=boolean  LogicDataType=fixdt(0, 8)  OutDataTypeStr=boolean
  Logical Operator5 : Logic  Operator=OR  Inputs=5  AllPortsSameDT=off  OutDataTypeMode=boolean  LogicDataType=fixdt(0, 8)  OutDataTypeStr=boolean
  Subsystem : Subsystem
  Subsystem1 : Subsystem
  Subsystem2 : Subsystem
  Subsystem3 : Subsystem
  Subsystem4 : Subsystem
  Switch{,1..4} (5 alike) : Switch  Criteria=u2 ~= 0  OutDataType=fixdt(1, 16)  OutScaling=2^0
  Valid : Outport  OutDataType=fixdt(1, 16)  OutScaling=2^0
  Out1 : Outport  Port=2  OutDataType=fixdt(1, 16)  OutScaling=2^0
  wires:
  Offset/1 -> Subsystem/1(In1), Subsystem1/1(In1), Subsystem2/1(In1), Subsystem3/1(In1), Subsystem4/1(In1)
  Compare To Constant/1 -> Subsystem/Enable, Logical Operator/1
  Size/1 -> Compare To Constant/1, Compare To Constant1/1, Compare To Constant2/1, Compare To Constant3/1, Compare To Constant4/1
  Compare To Constant1/1 -> Subsystem1/Enable, Logical Operator1/1
  Compare To Constant2/1 -> Subsystem2/Enable, Logical Operator2/1
  Compare To Constant3/1 -> Subsystem3/Enable, Logical Operator3/1
  Compare To Constant4/1 -> Subsystem4/Enable, Logical Operator4/1
  Subsystem/1(Valid) -> Logical Operator/2
  Subsystem1/1(Valid) -> Logical Operator1/2
  Subsystem2/1(Valid) -> Logical Operator2/2
  Subsystem3/1(Valid) -> Logical Operator3/2
  Subsystem4/1(Valid) -> Logical Operator4/2
  Logical Operator5/1 -> Valid/1
  Logical Operator/1 -> Logical Operator5/1, Switch/2
  Logical Operator4/1 -> Logical Operator5/5, Switch4/2
  Logical Operator3/1 -> Logical Operator5/4, Switch3/2
  Logical Operator2/1 -> Logical Operator5/3, Switch2/2
  Logical Operator1/1 -> Logical Operator5/2, Switch1/2
  Subsystem/2(Out) -> Switch/1
  Subsystem1/2(Out) -> Switch1/1
  Switch1/1 -> Switch/3
  Subsystem2/2(Out) -> Switch2/1
  Switch2/1 -> Switch1/3
  Switch/1 -> Out1/1
  Subsystem3/2(Out) -> Switch3/1
  Switch3/1 -> Switch2/3
  Switch4/1 -> Switch3/3
  Subsystem4/2(Out) -> Switch4/1
  Ground/1 -> Switch4/3

== system stm32f0_ccp_sensor/CCP Handler/Command Processing/UPLOAD/UPLOAD/UPLOAD/MEM_FLASH ==
  Offset : Inport  OutDataType=fixdt(1, 16)  OutScaling=2^0
  Size : Inport  Port=2  OutDataType=fixdt(1, 16)  OutScaling=2^0
  Enable : EnablePort
  Compare To Constant : simulink/Logic and Bit Operations/Compare To Constant  SystemSampleTime=-1  relop===  const=2  LogicOutDataTypeMode=uint8  ZeroCross=off
  Compare To Constant1 : simulink/Logic and Bit Operations/Compare To Constant  SystemSampleTime=-1  relop===  const=4  LogicOutDataTypeMode=uint8  ZeroCross=off
  Logical Operator : Logic  Operator=OR  AllPortsSameDT=off  OutDataTypeMode=boolean  LogicDataType=fixdt(0, 8)  OutDataTypeStr=boolean
  Read Flash 2 Byte : Subsystem  TreatAsAtomicUnit=on
  Read Flash 4 Byte : Subsystem  TreatAsAtomicUnit=on
  Switch : Switch  OutDataType=fixdt(1, 16)  OutScaling=2^0
  Valid : Outport  OutDataType=fixdt(1, 16)  OutScaling=2^0
  Out1 : Outport  Port=2  OutDataType=fixdt(1, 16)  OutScaling=2^0
  wires:
  Logical Operator/1 -> Valid/1
  Size/1 -> Compare To Constant/1, Compare To Constant1/1
  Compare To Constant/1 -> Read Flash 2 Byte/Enable, Logical Operator/1, Switch/2
  Compare To Constant1/1 -> Read Flash 4 Byte/Enable, Logical Operator/2
  Offset/1 -> Read Flash 2 Byte/1(Offset), Read Flash 4 Byte/1(In1)
  Read Flash 2 Byte/1(Out1) -> Switch/1
  Read Flash 4 Byte/1(Out1) -> Switch/3
  Switch/1 -> Out1/1

== system stm32f0_ccp_sensor/CCP Handler/Command Processing/UPLOAD/UPLOAD/UPLOAD/MEM_RO ==
  Offset : Inport  OutDataType=fixdt(1, 16)  OutScaling=2^0
  Size : Inport  Port=2  OutDataType=fixdt(1, 16)  OutScaling=2^0
  Enable : EnablePort
  Constant : Constant  OutDataTypeMode=uint8  OutDataType=fixdt(1, 16)  OutScaling=2^0  OutDataTypeStr=uint8
  Volatile Data Array Read : waijung_addon_module/Data Storage/Volatile Data Array Read  conf=Read  specificaddress=off  storagename=READ_DATA  memoryaddress=hex2dec('64000000')  storagetype=uint8  datasize=120*160*3  varname=VolatileDataArray_READ_DATA  datatype=uint8  datacount=5  variablesize=on  portpinstr=0  sampletime=inf  blockid=CCPHandlerCommandProcessingUPLOADUPLOADUPLOADMEM_ROVolatileDataArrayRead  inputporttype=[7 7]  inputportwidth=[1 1 ]  inputportlabel={'Offset','Size'}  outputporttype=[3]  outputportwidth=[5]  outputportlabel={'Data(5)'}  compat=0  optionstring="[\"READ_DATA\",\"uint8\",\"256\",\"VolatileDataArray_READ_DATA\",\"uint8_t\",\"uint8\",\"uint8_t\",\"5\",\"Param1\"]"
  Valid : Outport  OutDataType=fixdt(1, 16)  OutScaling=2^0
  Out1 : Outport  Port=2  OutDataType=fixdt(1, 16)  OutScaling=2^0
  wires:
  Offset/1 -> Volatile Data Array Read/1
  Volatile Data Array Read/1 -> Out1/1
  Size/1 -> Volatile Data Array Read/2
  Constant/1 -> Valid/1

== system stm32f0_ccp_sensor/CCP Handler/Command Processing/UPLOAD/UPLOAD/UPLOAD/MEM_RW ==
  Offset : Inport  OutDataType=fixdt(1, 16)  OutScaling=2^0
  Size : Inport  Port=2  OutDataType=fixdt(1, 16)  OutScaling=2^0
  Enable : EnablePort
  Constant : Constant  OutDataTypeMode=uint8  OutDataType=fixdt(1, 16)  OutScaling=2^0  OutDataTypeStr=uint8
  Volatile Data Array Read : waijung_addon_module/Data Storage/Volatile Data Array Read  conf=Read  specificaddress=off  storagename=CONTROL  memoryaddress=hex2dec('64000000')  storagetype=uint8  datasize=120*160*3  varname=VolatileDataArray_CONTROL  datatype=uint8  datacount=5  variablesize=on  portpinstr=0  sampletime=inf  blockid=CCPHandlerCommandProcessingUPLOADUPLOADUPLOADMEM_RWVolatileDataArrayRead  inputporttype=[7 7]  inputportwidth=[1 1 ]  inputportlabel={'Offset','Size'}  outputporttype=[3]  outputportwidth=[5]  outputportlabel={'Data(5)'}  compat=0  optionstring="[\"CONTROL\",\"uint8\",\"256\",\"VolatileDataArray_CONTROL\",\"uint8_t\",\"uint8\",\"uint8_t\",\"5\",\"Param1\"]"
  Valid : Outport  OutDataType=fixdt(1, 16)  OutScaling=2^0
  Out1 : Outport  Port=2  OutDataType=fixdt(1, 16)  OutScaling=2^0
  wires:
  Offset/1 -> Volatile Data Array Read/1
  Size/1 -> Volatile Data Array Read/2
  Volatile Data Array Read/1 -> Out1/1
  Constant/1 -> Valid/1

== system stm32f0_ccp_sensor/CCP Handler/Command Processing/UPLOAD/UPLOAD/UPLOAD/SLAVE_DEVICE_ID ==
  Offset : Inport  OutDataType=fixdt(1, 16)  OutScaling=2^0
  Size : Inport  Port=2  OutDataType=fixdt(1, 16)  OutScaling=2^0
  Enable : EnablePort
  Constant : Constant  OutDataTypeMode=uint8  OutDataType=fixdt(1, 16)  OutScaling=2^0  OutDataTypeStr=uint8
  Volatile Data Array Read : waijung_addon_module/Data Storage/Volatile Data Array Read  conf=Read  specificaddress=off  storagename=SLAVE_DEV_ID  memoryaddress=hex2dec('64000000')  storagetype=uint8  datasize=120*160*3  varname=VolatileDataArray_SLAVE_DEV_ID  datatype=uint8  datacount=5  variablesize=on  portpinstr=0  sampletime=inf  blockid=CCPHandlerCommandProcessingUPLOADUPLOADUPLOADSLAVE_DEVICE_IDVolatileDataArrayRead  inputporttype=[7 7]  inputportwidth=[1 1 ]  inputportlabel={'Offset','Size'}  outputporttype=[3]  outputportwidth=[5]  outputportlabel={'Data(5)'}  compat=0  optionstring="[\"SLAVE_DEV_ID\",\"uint8\",\"16\",\"VolatileDataArray_SLAVE_DEV_ID\",\"uint8_t\",\"uint8\",\"uint8_t\",\"5\",\"Param1\"]"
  Valid : Outport  OutDataType=fixdt(1, 16)  OutScaling=2^0
  Out1 : Outport  Port=2  OutDataType=fixdt(1, 16)  OutScaling=2^0
  wires:
  Offset/1 -> Volatile Data Array Read/1
  Size/1 -> Volatile Data Array Read/2
  Volatile Data Array Read/1 -> Out1/1
  Constant/1 -> Valid/1

== system stm32f0_ccp_sensor/CCP Handler/Command Processing/BUILD_CHKSUM/BUILD_CHKSUM Handler/Subsystem/While Iterator Subsystem/Subsystem ==
  In1 : Inport
  In2 : Inport  Port=2
  Enable : EnablePort
  CRC32 : waijung_crc_lib/CRC32  conf=<empty>  sampletime=-1  enablecustomportlabel=off  cinputportlabel=0  portpinstr=0  blockid=CCPHandlerCommandProcessingBUILD_CHKSUMBUILD_CHKSUMHandlerSubsystemWhileIteratorSubsystemSubsystemCRC32  inputporttype=[7 7]  inputportwidth=[1 -1]  inputportlabel={'Initial','Value'}  outputporttype=[7]  outputportwidth=[]  outputportlabel={'Output'}  compat=0  optionstring="[\"Param1\",\"Param1\"]"
  FLASH Read : stm32f0_flash_lib/FLASH Read  conf=Read  startaddress=0x8011000  pagesize=2k  datatype=uint32  enablestatus=off  sampletime=inf  filename='stm32f0_ccp_sensor.flash'  enablecustomportlabel=off  cinputportlabel=0  portpinstr=0  blockid=CCPHandlerCommandProcessingBUILD_CHKSUMBUILD_CHKSUMHandlerSubsystemWhileIteratorSubsystemSubsystemFLASHRead  inputporttype=[7]  inputportwidth=[]  inputportlabel={'Offset'}  outputporttype=[7]  outputportwidth=[]  outputportlabel={'Data'}  compat=0  optionstring="[\"8011000\",\"0\"]"
  Out1 : Outport
  wires:
  FLASH Read/1 -> CRC32/2
  In1/1 -> CRC32/1
  CRC32/1 -> Out1/1
  In2/1 -> FLASH Read/1

== system stm32f0_ccp_sensor/CCP Handler/Command Processing/CLEAR_MEMORY/CLEAR_MEMORY Handler/Flash Erase/While Iterator Subsystem/Subsystem ==
  Address : Inport
  Enable : EnablePort
  FLASH Erase : stm32f0_flash_lib/FLASH Erase  conf=Erase  startaddress=0x8011000  pagesize=2k  datatype=int32  enablestatus=on  sampletime=inf  filename='stm32f0_ccp_sensor.flash'  enablecustomportlabel=off  cinputportlabel=0  portpinstr=0  blockid=CCPHandlerCommandProcessingCLEAR_MEMORYCLEAR_MEMORYHandlerFlashEraseWhileIteratorSubsystemSubsystemFLASHErase  inputporttype=[7]  inputportwidth=[]  inputportlabel={'Page Offset'}  outputporttype=[3]  outputportwidth=[]  outputportlabel={'Status'}  compat=0  optionstring="[\"8011000\",\"0\"]"
  UART Tx : S-Function  FunctionName=stm32f0_uart  Parameters=conf,inputporttype,inputportwidth,outputporttype,outputportwidth,asciiheader,optionstring,headerstring,terminatorstring,asciidatatypestring,sampletime,blockid  EnableBusSupport=off  mask(stm32f0_uart){conf=Tx, uartmodule=1, baudrate=115200, databits=8, parity=No, stopbit=1, remaptxpin=A9, remaprxpin=A10, flowcontrol=None, remapctspin=Not used, remaprtspin=Not used, advanceoptions=off, rxbuffersize=64, txbuffersize=64, transfer=Non-Blocking, packetmode=Ascii, binheader='7E 7E', binterminator='03 03', porttype_double=0, porttype_single=0, porttype_int8=0, porttype_uint8=0, porttype_int16=0, porttype_uint16=0, porttype_int32=0, porttype_uint32=2, asciiformat='Erase 0x%X, sta=%u', rx_asciiterminator=CR (0x0D - "\r"), tx_asciiterminator=CRLF (0x0D 0x0A - "\r\n"), storagename=<empty>, varname=, asciiheader=Erase 0x%X, sta=%u\r\n, sampletime=inf, enablecustomportlabel=off, cinputportlabel=de, coutputportlabel=fff,ff,sdfsd, portpinstr=0, blockid=CCPHandlerCommandProcessingCLEAR_MEMORYCLEAR_MEMORYHandlerFlashEraseWhileIteratorSubsystemSubsystemUARTTx, inputporttype=[ -1 -1], inputportwidth=[], inputportlabel={ '%X' '%u'}, outputporttype=[], outputportwidth=[], outputportlabel={}, compat=0, optionstring=["1", "1", "A", "9", "1", "A", "10", "0", "*", "*", "0", "*", "*", "1", "1", "", "", "115200", "8", "No", "1", "None", "3", "2", "64", "64", "Ascii", "Non-Blocking", ""], headerstring=[], terminatorstring=["13","10"], asciidatatypestring=["uint32_t","uint32_t"], lastmodule=1}
      mask prompts: conf "Configuration"; uartmodule "UART Module"; baudrate "Baud rate (bps)"; databits "Data bits"; stopbit "Stop bit"; remaptxpin "Tx pin"; remaprxpin "Rx pin"; flowcontrol "Hardware flow control"; remapctspin "HW Flow control, CTS Pin"; remaprtspin "HW Flow control, RTS Pin"; advanceoptions "Advance options"; rxbuffersize "Rx buffer size (bytes)"; txbuffersize "Tx buffer size (bytes)"; packetmode "Packet mode"; binheader "Binary header (example: '7E 7E')"; binterminator "Binary terminator (example: '03 03')"; porttype_double "Number of data port, type DOUBLE"; porttype_single "Number of data port, type SINGLE"; porttype_int8 "Number of data port, type INT8"; porttype_uint8 "Number of data port, type UINT8"; porttype_int16 "Number of data port, type INT16"; porttype_uint16 "Number of data port, type UINT16"; porttype_int32 "Number of data port, type INT32"; porttype_uint32 "Number of data port, type UINT32"; asciiformat "Ascii format"; rx_asciiterminator "End of packet"; tx_asciiterminator "End of packet"; storagename "Buffer"; varname "Var name"; asciiheader "Ascii header (printf format)"; sampletime "Sample time (sec)"; enablecustomportlabel "Enable custom port labels (Ex. In1, In2, In3)"; cinputportlabel "Custom input port labels (Ex. In1, In2, In3)"; coutputportlabel "Custom output port labels (Ex. Out1, Out2, Out3)"; portpinstr "Port Pin String"; blockid "Block ID"; inputporttype "Input Port Type"; inputportwidth "Input Port Width"; inputportlabel "Input Port Label"; outputporttype "Output Port Type"; outputportwidth "Output Port Width"; outputportlabel "Output port label"; compat "Compatibility (Reserved for future use)"; optionstring "String(s) to be passed to TLC"; lastmodule "Last module selected"
      mask help:
      | UART Module
      |  - Select module corresponding to "UART Setup" block.
      | Transfer
      |  - Blocking: after write DMA buffer, the block wait until buffer empty.
      |  - Non-Blocking: the block will not wait for buffer empty.
      | Packet mode:
      |  - Ascii: sending data is ascii, Ascii format + End of packet.
      |  - Binary: sending data is binary format, Header + Data + Terminator
      |  - String Buffer: Volatile Data Storage variable name as sending data.
      | Ascii format:
      |  - %U, %I, %D, %O, %X, %u, %i, %d, %o, %x: Uint32
      |  - %E, %G, %F, %e, %g, %f: Single
      |  - %C, %c: Int8
      |  - %S, %s: (char *), this port is output of Volatile Data Storage Read block, which data type is string.
      mask init:
      | stm32f0_uart_callback('init');
      mask Help: web(fullfile(waijungdocroot,'stm32f0_uart_tx.htm'), '-browser')
      mask StyleString: popup(Setup|Tx|Rx),popup(1|2|3|4),edit,popup(8),popup(No|Odd|Even),popup(0.5|1|1.5|2),popup(Not used|A9|B6),popup(Not used|A10|B7),popup(None|RTS|CTS|RTS/CTS),popup(Not used|A11),popup(Not used|A12),checkbox,popup(16|32|64|128|256|512),popup(16|32|64|128|256|512),popup(Blocking|Non-Blocking),popup(Ascii|Binary|String Buffer),edit,edit,edit,edit,edit,edit,edit,edit,edit,edit,edit,popup(CR (0x0D - "\r")|LF (0x0A - "\n")|CRLF (0x0D 0x0A - "\r\n")),popup(CR (0x0D - "\r")|LF (0x0A - "\n")|CRLF (0x0D 0x0A - "\r\n")|None),popup(<empty>),edit,edit,edit,checkbox,edit,edit,edit,edit,edit,edit,edit,edit,edit,edit,edit,edit,edit,edit,edit,edit
      mask CallbackString: stm32f0_uart_callback('conf');|stm32f0_uart_callback('uartmodule');|||||||stm32f0_uart_callback('flowcontrol');|||stm32f0_uart_callback('advanceoptions');|||stm32f0_uart_callback('conf');|stm32f0_uart_callback('conf');|stm32f0_uart_callback('binheader');|stm32f0_uart_callback('binterminator');|||||||||stm32f0_uart_callback('asciiformat');|||stm32f0_uart_callback('storagename');|||stm32f0_uart_callback('sampletime');|stm32f0_uart_callback('enablecustomportlabel');|stm32f0_uart_callback('conf');|stm32f0_uart_callback('conf');||stm32f0_uart_callback('blockid');||||||||||||
      mask Display: text(0.95, 0.5, 'Module: USART1_Tx\nPacket: Ascii\nTransfer: Non-Blocking\nTs (sec): -1','ver','middle','hor','right'); port_label('input', 1,'%X'); port_label('input', 2,'%u');
  Sta : Outport  OutDataType=fixdt(1, 16)  OutScaling=2^0
  wires:
  Address/1 -> FLASH Erase/1, UART Tx/1
  FLASH Erase/1 -> Sta/1, UART Tx/2

== system stm32f0_ccp_sensor/CCP Handler/Command Processing/SHORT_UP/SHORT_UP Handler/UPLOAD/MEM_EEPROM/Subsystem ==
  In1 : Inport
  Enable : EnablePort
  Compare To Zero : simulink/Logic and Bit Operations/Compare To Zero  SystemSampleTime=-1  relop===  LogicOutDataTypeMode=uint8  ZeroCross=off
  Constant : Constant  Value=0  OutDataTypeMode=uint8  OutDataType=fixdt(1, 16)  OutScaling=2^0  OutDataTypeStr=uint8
  Constant1 : Constant  Value=hex2dec('A0')  OutDataTypeMode=uint8  OutDataType=fixdt(1, 16)  OutScaling=2^0  OutDataTypeStr=uint8
  Data Type Conversion : DataTypeConversion  OutDataType=fixdt(1, 16)  OutScaling=2^0
  Mux : Mux  Inputs=5
  Soft I2C Master Read/Write : waijung_soft_i2c_lib/Soft I2C Master Read//Write  conf=ReadWrite  targetname=stm32f0  module=1  transfer=Blocking  clk=100  timeout=25  sdapins={'A4','A6'}  sclpins='A5'  writecount=1  readcount=1  waittime=0  forcestop=off  portpinstr=0  sampletime=inf  blockid=CCPHandlerCommandProcessingSHORT_UPSHORT_UPHandlerUPLOADMEM_EEPROMSubsystemSoftI2CMasterReadWrite  inputporttype=[3 3]  inputportwidth=[]  inputportlabel={'SlvAddr' 'Wr0 (uint8)'}  outputporttype=[3 3 ]  outputportwidth=[1 1]  outputportlabel={'Status' 'Rd0 (uint8)'}  compat=0  optionstring="[\"1\",\"1\",\"1\",\"0\",\"off\",\"1\"]"
  Valid : Outport
  Out : Outport  Port=2  InitialOutput=[0 0 0 0 0]
  wires:
  Constant1/1 -> Soft I2C Master Read/Write/1
  Data Type Conversion/1 -> Soft I2C Master Read/Write/2
  Soft I2C Master Read/Write/1 -> Compare To Zero/1
  In1/1 -> Data Type Conversion/1
  Compare To Zero/1 -> Valid/1
  Soft I2C Master Read/Write/2 -> Mux/1
  Mux/1 -> Out/1
  Constant/1 -> Mux/3, Mux/2, Mux/4, Mux/5

== system stm32f0_ccp_sensor/CCP Handler/Command Processing/SHORT_UP/SHORT_UP Handler/UPLOAD/MEM_EEPROM/Subsystem1 ==
  In1 : Inport
  Enable : EnablePort
  Compare To Zero : simulink/Logic and Bit Operations/Compare To Zero  SystemSampleTime=-1  relop===  LogicOutDataTypeMode=uint8  ZeroCross=off
  Constant : Constant  Value=0  OutDataTypeMode=uint8  OutDataType=fixdt(1, 16)  OutScaling=2^0  OutDataTypeStr=uint8
  Constant1 : Constant  Value=hex2dec('A0')  OutDataTypeMode=uint8  OutDataType=fixdt(1, 16)  OutScaling=2^0  OutDataTypeStr=uint8
  Data Type Conversion : DataTypeConversion  OutDataType=fixdt(1, 16)  OutScaling=2^0
  Mux : Mux  Inputs=5
  Soft I2C Master Read/Write : waijung_soft_i2c_lib/Soft I2C Master Read//Write  conf=ReadWrite  targetname=stm32f0  module=1  transfer=Blocking  clk=100  timeout=25  sdapins={'A4','A6'}  sclpins='A5'  writecount=1  readcount=2  waittime=0  forcestop=off  portpinstr=0  sampletime=inf  blockid=CCPHandlerCommandProcessingSHORT_UPSHORT_UPHandlerUPLOADMEM_EEPROMSubsystem1SoftI2CMasterReadWrite  inputporttype=[3 3]  inputportwidth=[]  inputportlabel={'SlvAddr' 'Wr0 (uint8)'}  outputporttype="[3 3 3  ]"  outputportwidth=[1 1 1]  outputportlabel={'Status' 'Rd0 (uint8)' 'Rd1 (uint8)'}  compat=0  optionstring="[\"1\",\"1\",\"2\",\"0\",\"off\",\"1\"]"
  Valid : Outport
  Out : Outport  Port=2  InitialOutput=[0 0 0 0 0]
  wires:
  Mux/1 -> Out/1
  Soft I2C Master Read/Write/2 -> Mux/1
  Compare To Zero/1 -> Valid/1
  In1/1 -> Data Type Conversion/1
  Soft I2C Master Read/Write/1 -> Compare To Zero/1
  Data Type Conversion/1 -> Soft I2C Master Read/Write/2
  Constant1/1 -> Soft I2C Master Read/Write/1
  Soft I2C Master Read/Write/3 -> Mux/2
  Constant/1 -> Mux/4, Mux/3, Mux/5

== system stm32f0_ccp_sensor/CCP Handler/Command Processing/SHORT_UP/SHORT_UP Handler/UPLOAD/MEM_EEPROM/Subsystem2 ==
  In1 : Inport
  Enable : EnablePort
  Compare To Zero : simulink/Logic and Bit Operations/Compare To Zero  SystemSampleTime=-1  relop===  LogicOutDataTypeMode=uint8  ZeroCross=off
  Constant : Constant  Value=0  OutDataTypeMode=uint8  OutDataType=fixdt(1, 16)  OutScaling=2^0  OutDataTypeStr=uint8
  Constant1 : Constant  Value=hex2dec('A0')  OutDataTypeMode=uint8  OutDataType=fixdt(1, 16)  OutScaling=2^0  OutDataTypeStr=uint8
  Data Type Conversion : DataTypeConversion  OutDataType=fixdt(1, 16)  OutScaling=2^0
  Mux : Mux  Inputs=5
  Soft I2C Master Read/Write : waijung_soft_i2c_lib/Soft I2C Master Read//Write  conf=ReadWrite  targetname=stm32f0  module=1  transfer=Blocking  clk=100  timeout=25  sdapins={'A4','A6'}  sclpins='A5'  writecount=1  readcount=3  waittime=0  forcestop=off  portpinstr=0  sampletime=inf  blockid=CCPHandlerCommandProcessingSHORT_UPSHORT_UPHandlerUPLOADMEM_EEPROMSubsystem2SoftI2CMasterReadWrite  inputporttype=[3 3]  inputportwidth=[]  inputportlabel={'SlvAddr' 'Wr0 (uint8)'}  outputporttype="[3 3 3 3   ]"  outputportwidth=[1 1 1 1]  outputportlabel={'Status' 'Rd0 (uint8)' 'Rd1 (uint8)' 'Rd2 (uint8)'}  compat=0  optionstring="[\"1\",\"1\",\"3\",\"0\",\"off\",\"1\"]"
  Valid : Outport
  Out : Outport  Port=2  InitialOutput=[0 0 0 0 0]
  wires:
  Soft I2C Master Read/Write/3 -> Mux/2
  Constant1/1 -> Soft I2C Master Read/Write/1
  Data Type Conversion/1 -> Soft I2C Master Read/Write/2
  Soft I2C Master Read/Write/1 -> Compare To Zero/1
  In1/1 -> Data Type Conversion/1
  Compare To Zero/1 -> Valid/1
  Soft I2C Master Read/Write/2 -> Mux/1
  Mux/1 -> Out/1
  Soft I2C Master Read/Write/4 -> Mux/3
  Constant/1 -> Mux/4, Mux/5
